simulink model "power_PVarray_grid_det_LVRT"  (Simulink 8.7)
settings: Solver=FixedStepDiscrete  SolverMode=SingleTasking  StartTime=0.0  StopTime=1.666666  RelTol=1e-3
PreLoadFcn:
  | Ts_Power=1e-6;
  | Ts_Control=100e-6;
undefined symbols (not defined in the file): D1, Delta, DiscIntNeverNeededParam, sigbuilder_block
libraries: powerlib x30, powerlib_meascontrol x17, simulink x6, re_lib x1
(part 1 of 2)
Description:
  | Copyright 2008-2016 The MathWorks, Inc.
settings Model: Creator=MathWorks  LastModifiedBy=jherna4  SimulationMode=accelerator
settings DataIOCC: SignalLoggingSaveFormat=ModelDataLogs  SignalLogging=off  DSMLogging=off
settings OptimizationCC: ExpressionDepthLimit=2147483647
settings DebuggingCC: SolverPrmCheckMsg=warning  FcnCallInpInsideContextMsg=EnableAllAsWarning  StateNameClashWarn=warning
settings GRTTargetCC: CombineOutputUpdateFcns=off  GRTInterface=on
settings ConfigComp: CovModelRefEnable=off  CovSFcnEnable=off

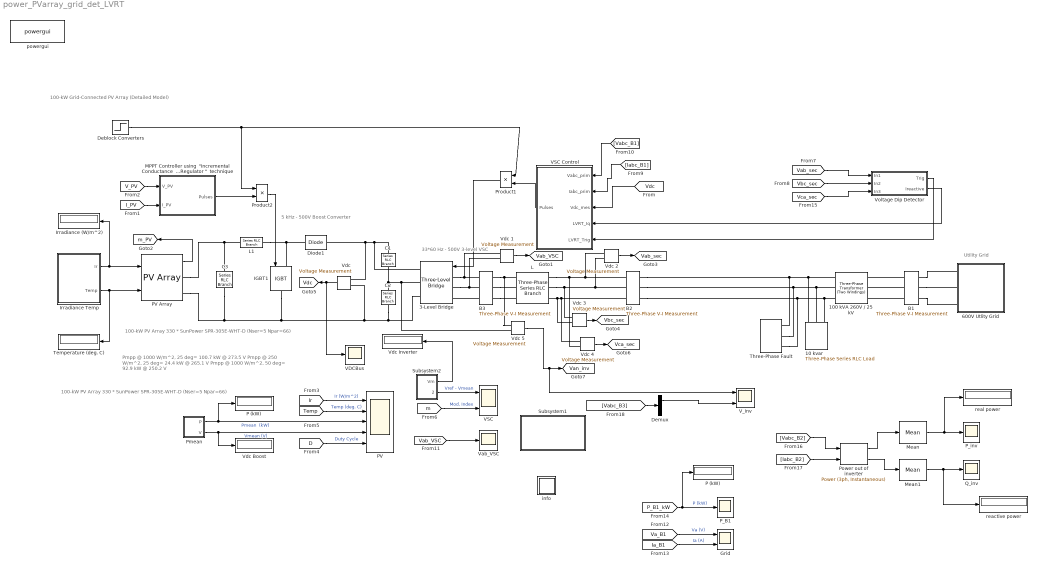
== system power_PVarray_grid_det_LVRT ==
  note: 5 kHz - 500V
      | Boost Converter
  note: 33*60 Hz - 500V
      | 3-level VSC
  note: 100-kW Grid-Connected PV Array (Detailed Model)
  note: Utility Grid
  note: Pmpp @ 1000 W/m^2, 25 deg= 100.7 kW @ 273.5 V
      | Pmpp @  250 W/m^2, 25 deg= 24.4  kW @ 265.1 V
      | Pmpp @ 1000 W/m^2, 50 deg= 92.9  kW @ 250.2 V
  note: 100-kW  PV Array
      | 330 * SunPower SPR-305E-WHT-D  (Nser=5 Npar=66)
  note: 100-kW  PV Array
      | 330 * SunPower SPR-305E-WHT-D  (Nser=5 Npar=66)
  10 kvar : powerlib/Elements/Three-Phase Series RLC Load  LConnTagsString=A|B|C  Configuration=Y (grounded)  NominalVoltage=240  Vabc=[1e3 1e3 1e3]  Vabcp=[1e3 1e3 1e3]  NominalFrequency=60  UnbalancedPower=off  ActivePower=10e3/100  InductivePower=0  CapacitivePower=10e3  Pabc=[10e3 9e3 11e3]  QLabc=[100 90 110]  QCabc=[100 90 110]  Pabcp=[10e3 9e3 11e3]  QLabcp=[100 90 110]  QCabcp=[100 90 110]  Measurements=None  LoadType=constant Z
  100 kVA 260V / 25 kV : powerlib/Elements/Three-Phase Transformer (Two Windings)  Winding1Connection=Yg  Winding2Connection=Delta (D1)  CoreType=Three single-phase transformers  SetSaturation=off  Hysteresis=off  DataFile='hysteresis'  SetInitialFlux=off  Measurements=None  UNITS=pu  NominalPower=[100e3 , 60 ]  Winding1=[ 25e3 , 0.001 , 0.03 ]  Winding2=[ 260 , 0.001 , 0.03 ]  Rm=500  Lm=500  L0=0.5  Saturation=[ 0,0 ; 0.0024,1.2 ; 1.0,1.52 ]  InitialFluxes=[ 0.8 , -0.8 , 0.7 ]  MoreParameters=off  BreakLoop=off  DataType=off  TransfoNumber=0
  3-Level Bridge : powerlib/Power Electronics/Three-Level Bridge  Arms=3  SnubberResistance=1e6  SbubberCapacitance=inf  Device=IGBT / Diodes  Ron=0.2e-3  ForwardVoltages="[  0  0 ]"  Measurements=None
  600V Utlity Grid : Subsystem
      mask Display: image(imread('grid.jpg'))
  B1 : powerlib/Measurements/Three-Phase V-I Measurement  VoltageMeasurement=phase-to-ground  SetLabelV=on  LabelV=Vabc_B1  Vpu=off  VpuLL=off  CurrentMeasurement=yes  SetLabelI=on  LabelI=Iabc_B1  Ipu=off  Pbase=100e6  Vbase=500e3  OutputType=Magnitude  PhasorSimulation=off  PSBequivalent=0
  B2 : powerlib/Measurements/Three-Phase V-I Measurement  VoltageMeasurement=phase-to-ground  SetLabelV=on  LabelV=Vabc_B2  Vpu=off  VpuLL=off  CurrentMeasurement=yes  SetLabelI=on  LabelI=Iabc_B2  Ipu=off  Pbase=100e6  Vbase=500e3  OutputType=Magnitude  PhasorSimulation=off  PSBequivalent=0
  B3 : powerlib/Measurements/Three-Phase V-I Measurement  VoltageMeasurement=phase-to-ground  SetLabelV=on  LabelV=Vabc_B3  Vpu=off  VpuLL=off  CurrentMeasurement=yes  SetLabelI=on  LabelI=Iabc_B3  Ipu=off  Pbase=100e6  Vbase=500e3  OutputType=Magnitude  PhasorSimulation=off  PSBequivalent=0
  C1 : powerlib/Elements/Series RLC Branch  LConnTagsString=__new0  RConnTagsString=__new0  BranchType=C  Resistance=1.0  Inductance=1.0  SetiL0=off  InitialCurrent=0  Capacitance=12000e-06  Setx0=off  InitialVoltage=0  Measurements=None
  C2 : powerlib/Elements/Series RLC Branch  LConnTagsString=__new0  RConnTagsString=__new0  BranchType=C  Resistance=1.0  Inductance=1.0  SetiL0=off  InitialCurrent=0  Capacitance=12000e-06  Setx0=off  InitialVoltage=0  Measurements=None
  C3 : powerlib/Elements/Series RLC Branch  LConnTagsString=__new0  RConnTagsString=__new0  BranchType=C  Resistance=1.0  Inductance=1.0  SetiL0=off  InitialCurrent=0  Capacitance=100e-6  Setx0=off  InitialVoltage=0  Measurements=Branch voltage
  Deblock Converters : Step  Time=0.05  SampleTime=0
  Demux : Demux  Outputs=3
  Diode1 : powerlib/Power Electronics/Diode  Ron=1e-4  Lon=0  Vf=0  IC=0  UseSnubber=off  Rs=inf  Cs=inf  Measurements=off
  Grid : Scope  NumInputPorts=2
  IGBT1 : powerlib/Power Electronics/IGBT  Ron=0.001  Lon=0  Vf=0  Tf=0  Tt=0  IC=0  Rs=1e5  Cs=inf  Measurements=off
  Irradiance (W/m^2) : Display
      settings: Format=bank  Decimation=1000
  Irradiance Temp : Subsystem  Tag=STV Subsys  LoadFcn=sigbuilder_block('load');  StartFcn=sigbuilder_block('start');  StopFcn=sigbuilder_block('stop');  ClipboardFcn=sigbuilder_block('clipboard');  mask(Sigbuilder block){}
      mask help: Sigbuilder GUI
      mask init:
      | if ~strcmp(get_param(bdroot(gcbh),'SimulationStatus'),'stopped') tuvar = sigbuilder_block('maskInit'); end
      settings: CopyFcn=sigbuilder_block('copy');  DeleteFcn=sigbuilder_block('delete');  ModelCloseFcn=sigbuilder_block('modelClose');  PreSaveFcn=sigbuilder_block('preSave');  PauseFcn=sigbuilder_block('pause')  ContinueFcn=sigbuilder_block('continue')  NameChangeFcn=sigbuilder_block('namechange');  OpenFcn=sigbuilder_block('open',[6 30 1428 682.5 ]);  CloseFcn=sigbuilder_block('close');
      mask Display: plot(0,0,100,100,[10,10,40,40,10],[80,20,20,80,80],[40,10],[50,50], [40,27,10],[65,72,56],[40,25,25,10],[28,28,43,43]);
  L : powerlib/Elements/Three-Phase Series RLC Branch  LConnTagsString=A|B|C  RConnTagsString=A|B|C  BranchType=RL  Resistance=500e-6*377/50/2  Inductance=500e-6/2  Capacitance=inf  Measurements=None
  L1 : powerlib/Elements/Series RLC Branch  LConnTagsString=__new0  RConnTagsString=__new0  BranchType=RL  Resistance=0.005  Inductance=5e-3  SetiL0=off  InitialCurrent=0  Capacitance=1e-6  Setx0=off  InitialVoltage=0  Measurements=None
  "MPPT Controller using  \"Incremental Conductance  + Integral Regulator \"  technique " : Subsystem  mask(Boost Control - MPPT){fc=5000, T_MPPT=200e-6, Dinit=0.5}
      mask prompts: fc "PWM switching frequency (Hz)"; T_MPPT "Time window used by MPPT control (s)"; Dinit "Initial value of duty cycle"
  Mean : powerlib_meascontrol/Measurements/Mean  Freq=60  Vinit=0  Ts=Ts_Power
  Mean1 : powerlib_meascontrol/Measurements/Mean  Freq=60  Vinit=0  Ts=Ts_Power
  P (kW) : Display
      settings: Format=bank  Decimation=2000
  "P (kW) " : Display
      settings: Format=bank  Decimation=2000
  PV : Scope  NumInputPorts=5
  PV Array : re_lib/Solar/PV Array  Npar=66  Nser=5  PlotType=array @ 1000 W/m2 & specified temperatures  S_vec="[ 1000  250 ]"  Temp_C_vec="[0 25 50  ]"  ModuleName=SunPower SPR-305E-WHT-D  PlotWhenSelected=off  Pm=305.226  Ncell=96  Voc=64.2  Isc=5.96  Vm=54.7  Im=5.58  beta_Voc_pc=-0.27269  alpha_Isc_pc=0.061745  beta_Voc=-0.17507  alpha_Isc=0.00368  IL=6.0092  I0=6.3014e-12  nI=0.94504  Rsh=269.5934  Rs=0.37152  BAL=on  Tc=Tc  Tfilter=Tc
  P_B1 : Scope
  P_inv : Scope
  Pmean : Subsystem
  Power out of inverter : powerlib_meascontrol/Measurements/Power (3ph, Instantaneous)
  Product1 : Product  RndMeth=Zero
  Product2 : Product  RndMeth=Zero
  Q_inv : Scope
  Subsystem1 : Subsystem
      mask Display: disp('Open this block\nto display additional \nscopes & measurements')
  Subsystem2 : Subsystem
  Temperature (deg. C) : Display
      settings: Format=bank  Decimation=1000
  Three-Phase Fault : powerlib/Elements/Three-Phase Fault  InitialStates=0  FaultA=on  FaultB=on  FaultC=on  GroundFault=on  SwitchTimes="[90/60  100/60]"  External=off  SwitchStatus=NaN  FaultResistance=0.025  GroundResistance=0.01  SnubberResistance=1e6  SnubberCapacitance=inf  Measurements=None
  VDCBus : Scope
  VSC : Scope  NumInputPorts=2
  VSC Control : Subsystem  mask(VSC Main Controller){nom=[ 100e3  60 ], Vnom=[ 25e3 260 ], Vnom_dc=500, RLxfo=[0.002  0.06 ], RLchoke=[2e-3  250e-6  ], K_VDCreg=[7  800], K_Ireg=[0.3 20], Ts=Ts_Control}
      mask prompts: nom "Nominal power and frequency [ Pnom(VA)  Fnom(Hz) ]:"; Vnom "Nominal primary and secondary voltages (Vrms LL) [ Vnom_prim   Vnom_sec ]:"; Vnom_dc "Nominal DC bus voltage (V):"; RLxfo "Total transformer leakage impedance (pu/Pnom) [ Rxfo  Lxf ]"; RLchoke "Choke impedance [ R(ohm) L(H) ]"; K_VDCreg "VDC regultator gains [ Kp  Ki ]:"; K_Ireg "Current regulator gains [ Kp  Ki ]:"; Ts "Sample time"
      mask init:
      | Pnom=nom(1);
      | Fnom=nom(2);
      | Vnom_prim=Vnom(1);
      | Vnom_sec=Vnom(2);
      | Zbase=Vnom_sec^2/Pnom;
      | Rtot_pu=RLxfo(1) + RLchoke(1)/Zbase;
      | Ltot_pu=RLxfo(2) + RLchoke(2)/(Zbase/(2*pi*Fnom));
      | Kp_VDCreg=K_VDCreg(1);
      | Ki_VDCreg=K_VDCreg(2);
      | Kp_Ireg=K_Ireg(1);
      | Ki_Ireg=K_Ireg(2);
      | Vdc_ref=Vnom_dc;
      | % Used to determine initial value of Boost Control (MPPT)
      | assignin('base','Vdc_ref_Inv',Vdc_ref);
  "V_inv " : Scope  NumInputPorts=2
  Vab_VSC : Scope
  Vdc {,1..5} (6 alike) : powerlib/Measurements/Voltage Measurement  Tag=PoWeRsYsTeMmEaSuReMeNt  PhasorSimulation=off  OutputType=Magnitude  PSBequivalent=0
  Vdc Boost : Display
      settings: Format=bank  Decimation=2000
  Vdc Inverter : Display
      settings: Format=bank  Decimation=2000
  Voltage Dip Detector : Subsystem
  info : Subsystem
      settings: OpenFcn=showdemo(bdroot(gcb))
      mask Display: disp('?')
  powergui : powerlib/powergui  Priority=1  SimulationMode=Discrete  SolverType=Tustin/Backward Euler (TBE)  SampleTime=Ts_Power  frequency=60  SPID=off  DisableSnubberDevices=off  DisableRonSwitches=off  DisableVfSwitches=off  SwTol=0  DisplayEquations=off  Interpol=off  ExternalGateDelay=off  methode=off  Ts=0  FunctionMessages=off  echomessages=off  HookPort=off  EnableUseOfTLC=off  x0status=blocks  frequencyindice=0  Pbase=100e6  ErrMax=1e-4  Iterations=50  UnitsV=kV  UnitsW=MW  buscounter=0  RestoreLinks=warning  ResistiveCurrentMeasurement=off  Frange=[0:2:500]  Ylog=off  Xlog=on  ShowGrid=off  save=off  variable=ZData  structure=0  ZoomFFT=on  StartTime=0.0  cycles=1  DisplayStyle=1  fundamental=60  FreqAxis=off  MaxFrequency=1000  frequencyindicesteady=1  RmsSteady=1  display=off
  reactive power : Display
  real power : Display
  tag scope: Vab_VSC=global, Vab_sec=global, Van_inv=global, Vbc_sec=global, Vca_sec=global, Vdc=global, m_PV=global
  wires:
  "Vdc "/1 -> VDCBus/1, [Vdc]
  Product2/1 -> IGBT1/1
  "MPPT Controller using  \"Incremental Conductance  + Integral Regulator \"  technique "/1(Pulses) -> Product2/2
  Deblock Converters/1 -> Product2/1, Product1/1
  [Vabc_B1] -> VSC Control/1(Vabc_prim)
  [Iabc_B1] -> VSC Control/2(Iabc_prim)
  [Vdc] -> VSC Control/3(Vdc_mes)
  VSC Control/1(Pulses) -> Product1/2
  Product1/1 -> 3-Level Bridge/1
  [I_PV] -> "MPPT Controller using  \"Incremental Conductance  + Integral Regulator \"  technique "/2(I_PV)
  [V_PV] -> "MPPT Controller using  \"Incremental Conductance  + Integral Regulator \"  technique "/1(V_PV)
  Pmean/1(P) -> "P (kW) "/1, PV/3  "Pmean  (kW)"
  [m] -> VSC/2  "Mod. Index"
  Vdc 1/1 -> [Vab_VSC]
  [Vab_VSC] -> Vab_VSC/1
  [Ia_B1] -> Grid/2  "Ia (A)"
  [Va_B1] -> Grid/1  "Va (V)"
  [P_B1_kW] -> P_B1/1, P (kW)/1  "P (kW)"
  Pmean/2(V) -> Vdc Boost/1, PV/4  "Vmean (V)"
  Subsystem2/2(VrVm) -> VSC/1  "Vref - Vmean"
  Subsystem2/1(Vm) -> Vdc Inverter/1
  PV Array/1 -> [m_PV]
  Irradiance Temp/1(Ir) -> PV Array/1, Irradiance (W/m^2)/1
  Irradiance Temp/2(Temp) -> PV Array/2, Temperature (deg. C)/1
  [D] -> PV/5  "Duty Cycle"
  [Temp] -> PV/2  "Temp (deg. C)"
  [Ir] -> PV/1  "Ir (W/m^2)"
  Vdc 2/1 -> [Vab_sec]
  Vdc 3/1 -> [Vbc_sec]
  Vdc 4/1 -> [Vca_sec]
  [Vab_sec] -> Voltage Dip Detector/1(In1)
  [Vbc_sec] -> Voltage Dip Detector/2(In2)
  [Vca_sec] -> Voltage Dip Detector/3(In3)
  [Vabc_B2] -> Power out of inverter/1
  [Iabc_B2] -> Power out of inverter/2
  Power out of inverter/1 -> Mean/1
  Power out of inverter/2 -> Mean1/1
  Mean/1 -> real power/1, P_inv/1
  Mean1/1 -> reactive power/1, Q_inv/1
  Voltage Dip Detector/1(Trig) -> VSC Control/5(LVRT_Trig)
  Voltage Dip Detector/2(Ireactive) -> VSC Control/4(LVRT_Iq)
  Vdc 5/1 -> "V_inv "/1, [Van_inv]
  [Vabc_B3] -> Demux/1
  Demux/1 -> "V_inv "/2
  connections:
  C1/LConn1 -- 3-Level Bridge/RConn1 -- Diode1/RConn1 -- "Vdc "/LConn1
  L1/RConn1 -- Diode1/LConn1 -- IGBT1/LConn1
  3-Level Bridge/RConn3 -- C2/RConn1 -- "Vdc "/LConn2 -- IGBT1/RConn1 -- PV Array/RConn2 -- C3/RConn1
  3-Level Bridge/LConn1 -- B3/LConn1 -- Vdc 1/LConn1
  3-Level Bridge/LConn2 -- B3/LConn2 -- Vdc 1/LConn2
  L/RConn1 -- B2/LConn1 -- Vdc 2/LConn1 -- Vdc 4/LConn2
  L/RConn2 -- B2/LConn2 -- Vdc 2/LConn2 -- Vdc 3/LConn1
  Three-Phase Fault/LConn3 -- B2/RConn3 -- 100 kVA 260V / 25 kV/RConn3 -- 10 kvar/LConn3
  B1/LConn1 -- 100 kVA 260V / 25 kV/LConn1
  B1/LConn2 -- 100 kVA 260V / 25 kV/LConn2
  B1/LConn3 -- 100 kVA 260V / 25 kV/LConn3
  C2/LConn1 -- Vdc 5/LConn2 -- 3-Level Bridge/RConn2 -- C1/RConn1
  C3/LConn1 -- PV Array/RConn1 -- L1/LConn1
  B1/RConn2 -- 600V Utlity Grid/LConn2
  B1/RConn1 -- 600V Utlity Grid/LConn1
  B1/RConn3 -- 600V Utlity Grid/LConn3
  Three-Phase Fault/LConn1 -- 100 kVA 260V / 25 kV/RConn1 -- 10 kvar/LConn1 -- B2/RConn1
  Three-Phase Fault/LConn2 -- B2/RConn2 -- 100 kVA 260V / 25 kV/RConn2 -- 10 kvar/LConn2
  L/RConn3 -- B2/LConn3 -- Vdc 4/LConn1 -- Vdc 3/LConn2
  B3/RConn1 -- Vdc 5/LConn1 -- L/LConn1
  B3/RConn2 -- L/LConn2
  B3/LConn3 -- 3-Level Bridge/LConn3
  B3/RConn3 -- L/LConn3

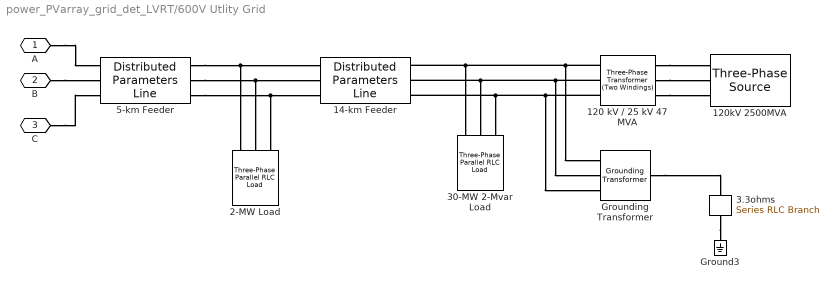
== system power_PVarray_grid_det_LVRT/600V Utlity Grid ==
  120 kV / 25 kV 47 MVA : powerlib/Elements/Three-Phase Transformer (Two Windings)  Winding1Connection=Yg  Winding2Connection=Delta (D1)  CoreType=Three single-phase transformers  SetSaturation=off  Hysteresis=off  DataFile='basic_model'  SetInitialFlux=off  Measurements=None  UNITS=pu  NominalPower=[47e6 60 ]  Winding1="[ 120e3  0.08/30   0.08 ]"  Winding2="[ 25e3  0.08/30  0.08]"  Rm=500  Lm=500  L0=0.5  Saturation="[ 0,0  ;  0.005,1.2  ;  1.0,1.4 ]"  InitialFluxes=[ 0.8 , -0.8 , 0.7 ]  MoreParameters=off  BreakLoop=off  DataType=off  TransfoNumber=0
  120kV 2500MVA : powerlib/Electrical Sources/Three-Phase Source  InternalConnection=Yg  VoltagePhases=off  Voltage=120e3  PhaseAngle=0  Voltage_phases=[25e3 25e3 25e3]/sqrt(3)  PhaseAngles_phases=[0 -120 +120]  Frequency=60  NonIdealSource=on  SpecifyImpedance=on  Resistance=0.8929  Inductance=16.58e-3  ShortCircuitLevel=2500e6  BaseVoltage=120e3  XRratio=7  BusType=swing  Pref=0  Qref=0  Prefabc=[10e3, 10e3, 10e3]  Qrefabc=[0, 0, 0]  Qmin=-inf  Qmax=inf
  14-km Feeder : powerlib/Elements/Distributed Parameters Line  Phases=3  Frequency=60  Resistance=[0.1153 0.413]  Inductance=[1.05e-3 3.32e-3]  Capacitance=[11.33e-009 5.01e-009]  Length=14  x1=[-5.8e-05 -3.07268501543022e-09 0 0;-5.7e-05 -3.07225125790422e-09 0 0;-5.6e-05 -3.07181706374279e-09 0 0;-5.5e-05 -3.07138243300766e-09 0 0;-5.4e-05 -3.07094736576058e-09 0 0;-5.3e-05 -3.0705118620634e-09 0 0;-5.2e-05 -3.070075921978e-09 0 0;-5.1e-05 -3.06963954556634e-09 0 0;-5e-05 -3.06920273289045e-09 0 0;-4.9e-05 -3.0687654840124e-09 -3790.73537143814 -24061.4134110798;-4.8e-05 -3.06832779899434e-09 -3781.66416312612 -24062.8407747816;-4.7e-05 -3.06788967789847e-09 -3772.59241735528 -24064.264718617;-4.6e-05 -3.06745112078705e-09 -3763.52013541492 -24065.6852423838;-4.5e-05 -3.06701212772242e-09 -3754.44731859442 -24067.10234588;-4.4e-05 -3.06657269876697e-09 -3745.37396818323 -24068.5160289042;-4.3e-05 -3.06613283398315e-09 -3736.30008547086 -24069.9262912555;-4.2e-05 -3.06569253343347e-09 -3727.22567174693 -24071.3331327335;-4.1e-05 -3.06525179718052e-09 -3718.15072830111 -24072.7365531382;-4e-05 -3.06481062528692e-09 -3709.07525642314 -24074.1365522702;-3.9e-05 -3.06436901781538e-09 -3699.99925740287 -24075.5331299305;-3.8e-05 -3.06392697482867e-09 -3690.92273253018 -24076.9262859206;-3.7e-05 -3.0634844963896e-09 -3681.84568309506 -24078.3160200426;-3.6e-05 -3.06304158256106e-09 -3672.76811038756 -24079.7023320988;-3.5e-05 -3.06259823340601e-09 -3663.6900156978 -24081.0852218923;-3.4e-05 -3.06215444898744e-09 -3654.61140031598 -24082.4646892266;-3.3e-05 -3.06171022936843e-09 -3645.53226553238 -24083.8407339055;-3.2e-05 -3.06126557461212e-09 -3636.45261263734 -24085.2133557336;-3.1e-05 -3.0608204847817e-09 -3627.37244292129 -24086.5825545157;-3e-05 -3.06037495994043e-09 -3618.29175767471 -24087.9483300573;-2.9e-05 -3.05992900015163e-09 -3609.21055818818 -24089.3106821641;-2.8e-05 -3.05948260547867e-09 -3600.12884575234 -24090.6696106428;-2.7e-05 -3.059035775985e-09 -3591.04662165791 -24092.0251153;-2.6e-05 -3.05858851173413e-09 -3581.96388719566 -24093.3771959431;-2.5e-05 -3.05814081278961e-09 -3572.88064365646 -24094.72585238;-2.4e-05 -3.05769267921509e-09 -3563.79689233123 -24096.071084419;-2.3e-05 -3.05724411107425e-09 -3554.712634511 -24097.412891869;-2.2e-05 -3.05679510843083e-09 -3545.62787148682 -24098.7512745391;-2.1e-05 -3.05634567134866e-09 -3536.54260454984 -24100.0862322393;-2e-05 -3.05589579989161e-09 -3527.45683499129 -24101.4177647797;-1.9e-05 -3.05544549412361e-09 -3518.37056410246 -24102.7458719712;-1.8e-05 -3.05499475410866e-09 -3509.2837931747 -24104.0705536249;-1.7e-05 -3.05454357991083e-09 -3500.19652349946 -24105.3918095526;-1.6e-05 -3.05409197159424e-09 -3491.10875636822 -24106.7096395666;-1.5e-05 -3.05363992922306e-09 -3482.02049307258 -24108.0240434795;-1.4e-05 -3.05318745286155e-09 -3472.93173490417 -24109.3350211046;-1.3e-05 -3.05273454257401e-09 -3463.8424831547 -24110.6425722555;-1.2e-05 -3.05228119842481e-09 -3454.75273911597 -24111.9466967463;-1.1e-05 -3.05182742047839e-09 -3445.66250407983 -24113.2473943918;-1e-05 -3.05137320879922e-09 -3436.5717793382 -24114.5446650071;-9e-06 -3.05091856345187e-09 -3427.48056618309 -24115.8385084078;-8e-06 -3.05046348450096e-09 -3418.38886590654 -24117.12892441;-7e-06 -3.05000797201115e-09 -3409.2966798007 -24118.4159128303;-6e-06 -3.04955202604718e-09 -3400.20400915777 -24119.6994734858;-5e-06 -3.04909564667387e-09 -3391.11085527002 -24120.9796061942;-4e-06 -3.04863883395606e-09 -3382.01721942979 -24122.2563107734;-3e-06 -3.04818158795869e-09 -3372.92310292949 -24123.529587042;-2e-06 -3.04772390874673e-09 -3363.82850706159 -24124.7994348191;-1e-06 -3.04726579638523e-09 -3354.73343311865 -24126.0658539241]  x2=[-5.8e-05 -3.21435514712151e-09 0 0;-5.7e-05 -3.21386287362357e-09 0 0;-5.6e-05 -3.21337014336404e-09 0 0;-5.5e-05 -3.21287695641295e-09 0 0;-5.4e-05 -3.21238331284039e-09 0 0;-5.3e-05 -3.21188921271652e-09 0 0;-5.2e-05 -3.21139465611156e-09 0 0;-5.1e-05 -3.2108996430958e-09 0 0;-5e-05 -3.2104041737396e-09 0 0;-4.9e-05 -3.20990824811336e-09 -3379.39243175417 -24244.0512711511;-4.8e-05 -3.20941186628758e-09 -3370.25239982314 -24245.3235492432;-4.7e-05 -3.20891502833279e-09 -3361.11188890409 -24246.5923815342;-4.6e-05 -3.20841773431962e-09 -3351.97090029607 -24247.8577678435;-4.5e-05 -3.20791998431873e-09 -3342.82943529824 -24249.1197079916;-4.4e-05 -3.20742177840087e-09 -3333.6874952098 -24250.3782017989;-4.3e-05 -3.20692311663684e-09 -3324.54508133001 -24251.6332490867;-4.2e-05 -3.20642399909752e-09 -3315.40219495823 -24252.8848496765;-4.1e-05 -3.20592442585384e-09 -3306.25883739385 -24254.1330033905;-4e-05 -3.2054243969768e-09 -3297.11500993636 -24255.3777100513;-3.9e-05 -3.20492391253747e-09 -3287.9707138853 -24256.618969482;-3.8e-05 -3.20442297260698e-09 -3278.82595054026 -24257.8567815062;-3.7e-05 -3.20392157725652e-09 -3269.68072120094 -24259.0911459479;-3.6e-05 -3.20341972655734e-09 -3260.53502716707 -24260.3220626318;-3.5e-05 -3.20291742058079e-09 -3251.38886973846 -24261.5495313829;-3.4e-05 -3.20241465939823e-09 -3242.24225021497 -24262.7735520267;-3.3e-05 -3.20191144308114e-09 -3233.09516989656 -24263.9941243892;-3.2e-05 -3.20140777170102e-09 -3223.94763008321 -24265.2112482971;-3.1e-05 -3.20090364532946e-09 -3214.79963207501 -24266.4249235773;-3e-05 -3.2003990640381e-09 -3205.65117717209 -24267.6351500573;-2.9e-05 -3.19989402789867e-09 -3196.50226667464 -24268.8419275652;-2.8e-05 -3.19938853698293e-09 -3187.35290188293 -24270.0452559294;-2.7e-05 -3.19888259136273e-09 -3178.2030840973 -24271.2451349789;-2.6e-05 -3.19837619110997e-09 -3169.05281461812 -24272.4415645432;-2.5e-05 -3.19786933629662e-09 -3159.90209474587 -24273.6345444522;-2.4e-05 -3.19736202699473e-09 -3150.75092578105 -24274.8240745364;-2.3e-05 -3.19685426327638e-09 -3141.59930902426 -24276.0101546268;-2.2e-05 -3.19634604521375e-09 -3132.44724577615 -24277.1927845547;-2.1e-05 -3.19583737287906e-09 -3123.29473733743 -24278.371964152;-2e-05 -3.19532824634461e-09 -3114.14178500886 -24279.5476932513;-1.9e-05 -3.19481866568275e-09 -3104.9883900913 -24280.7199716854;-1.8e-05 -3.19430863096591e-09 -3095.83455388564 -24281.8887992877;-1.7e-05 -3.19379814226657e-09 -3086.68027769285 -24283.054175892;-1.6e-05 -3.19328719965729e-09 -3077.52556281396 -24284.2161013328;-1.5e-05 -3.19277580321069e-09 -3068.37041055005 -24285.3745754449;-1.4e-05 -3.19226395299944e-09 -3059.21482220227 -24286.5295980637;-1.3e-05 -3.19175164909629e-09 -3050.05879907184 -24287.6811690249;-1.2e-05 -3.19123889157404e-09 -3040.90234246004 -24288.8292881651;-1.1e-05 -3.19072568050559e-09 -3031.74545366819 -24289.9739553209;-1e-05 -3.19021201596385e-09 -3022.5881339977 -24291.1151703297;-9e-06 -3.18969789802184e-09 -3013.43038475003 -24292.2529330293;-8e-06 -3.18918332675262e-09 -3004.2722072267 -24293.387243258;-7e-06 -3.18866830222933e-09 -2995.11360272928 -24294.5181008546;-6e-06 -3.18815282452516e-09 -2985.95457255943 -24295.6455056583;-5e-06 -3.18763689371337e-09 -2976.79511801884 -24296.769457509;-4e-06 -3.18712050986728e-09 -2967.63524040928 -24297.8899562469;-3e-06 -3.1866036730603e-09 -2958.47494103256 -24299.0070017128;-2e-06 -3.18608638336587e-09 -2949.31422119058 -24300.1205937478;-1e-06 -3.18556864085751e-09 -2940.15308218527 -24301.2307321938]  x3=[-5.8e-05 -1.41208605432097e-11 0 0;-5.7e-05 -1.41218449859166e-11 0 0;-5.6e-05 -1.41228274215944e-11 0 0;-5.5e-05 -1.41238078501035e-11 0 0;-5.4e-05 -1.41247862713045e-11 0 0;-5.3e-05 -1.41257626850583e-11 0 0;-5.2e-05 -1.41267370912263e-11 0 0;-5.1e-05 -1.41277094896699e-11 0 0;-5e-05 -1.41286798802508e-11 0 0;-4.9e-05 -1.41296482628313e-11 -23.5442852816691 -155.681480348964;-4.8e-05 -1.41306146372736e-11 -23.4855930745795 -155.69034527229;-4.7e-05 -1.41315790034405e-11 -23.4268975296635 -155.699188068545;-4.6e-05 -1.41325413611948e-11 -23.3681986552628 -155.708008736473;-4.5e-05 -1.41335017103998e-11 -23.30949645972 -155.716807274821;-4.4e-05 -1.4134460050919e-11 -23.2507909513778 -155.725583682338;-4.3e-05 -1.41354163826162e-11 -23.1920821385798 -155.734337957776;-4.2e-05 -1.41363707053555e-11 -23.1333700296696 -155.743070099892;-4.1e-05 -1.41373230190013e-11 -23.0746546329917 -155.751780107444;-4e-05 -1.41382733234182e-11 -23.0159359568907 -155.760467979195;-3.9e-05 -1.41392216184711e-11 -22.9572140097119 -155.76913371391;-3.8e-05 -1.41401679040253e-11 -22.8984887998011 -155.777777310356;-3.7e-05 -1.41411121799463e-11 -22.8397603355043 -155.786398767307;-3.6e-05 -1.41420544460999e-11 -22.7810286251682 -155.794998083535;-3.5e-05 -1.41429947023522e-11 -22.7222936771398 -155.803575257821;-3.4e-05 -1.41439329485695e-11 -22.6635554997668 -155.812130288943;-3.3e-05 -1.41448691846185e-11 -22.6048141013971 -155.820663175687;-3.2e-05 -1.41458034103661e-11 -22.5460694903792 -155.829173916839;-3.1e-05 -1.41467356256796e-11 -22.4873216750621 -155.837662511191;-3e-05 -1.41476658304265e-11 -22.428570663795 -155.846128957535;-2.9e-05 -1.41485940244745e-11 -22.3698164649278 -155.854573254669;-2.8e-05 -1.41495202076918e-11 -22.3110590868108 -155.862995401392;-2.7e-05 -1.41504443799467e-11 -22.2522985377947 -155.871395396508;-2.6e-05 -1.41513665411079e-11 -22.1935348262308 -155.879773238822;-2.5e-05 -1.41522866910443e-11 -22.1347679604706 -155.888128927143;-2.4e-05 -1.41532048296251e-11 -22.0759979488662 -155.896462460285;-2.3e-05 -1.41541209567199e-11 -22.0172247997702 -155.904773837063;-2.2e-05 -1.41550350721984e-11 -21.9584485215356 -155.913063056296;-2.1e-05 -1.41559471759308e-11 -21.8996691225157 -155.921330116806;-2e-05 -1.41568572677874e-11 -21.8408866110644 -155.929575017417;-1.9e-05 -1.41577653476388e-11 -21.782100995536 -155.937797756958;-1.8e-05 -1.41586714153561e-11 -21.7233122842853 -155.94599833426;-1.7e-05 -1.41595754708103e-11 -21.6645204856674 -155.954176748158;-1.6e-05 -1.41604775138731e-11 -21.6057256080381 -155.962332997489;-1.5e-05 -1.41613775444163e-11 -21.5469276597533 -155.970467081095;-1.4e-05 -1.41622755623119e-11 -21.4881266491695 -155.978578997819;-1.3e-05 -1.41631715674323e-11 -21.4293225846437 -155.986668746508;-1.2e-05 -1.41640655596501e-11 -21.3705154745333 -155.994736326013;-1.1e-05 -1.41649575388384e-11 -21.311705327196 -156.002781735187;-1e-05 -1.41658475048702e-11 -21.2528921509901 -156.010804972886;-9e-06 -1.41667354576193e-11 -21.1940759542742 -156.018806037971;-8e-06 -1.41676213969592e-11 -21.1352567454075 -156.026784929304;-7e-06 -1.41685053227642e-11 -21.0764345327495 -156.034741645751;-6e-06 -1.41693872349087e-11 -21.0176093246601 -156.042676186182;-5e-06 -1.41702671332672e-11 -20.9587811294996 -156.050588549468;-4e-06 -1.41711450177147e-11 -20.899949955629 -156.058478734485;-3e-06 -1.41720208881264e-11 -20.8411158114093 -156.066346740112;-2e-06 -1.4172894744378e-11 -20.7822787052023 -156.074192565231;-1e-06 -1.41737665863451e-11 -20.72343864537 -156.082016208726]  x4=[-5.8e-05 6.64255961640974e-12 0 0;-5.7e-05 6.64505542156155e-12 0 0;-5.6e-05 6.64755028230278e-12 0 0;-5.5e-05 6.65004419827886e-12 0 0;-5.4e-05 6.65253716913536e-12 0 0;-5.3e-05 6.65502919451797e-12 0 0;-5.2e-05 6.6575202740725e-12 0 0;-5.1e-05 6.66001040744494e-12 0 0;-5e-05 6.66249959428136e-12 0 0;-4.9e-05 6.66498783422801e-12 -1.3558131993987 -2.1529826150637;-4.8e-05 6.66747512693124e-12 -1.35500144774826 -2.1534935915926;-4.7e-05 6.66996147203756e-12 -1.3541895035219 -2.15400426206203;-4.6e-05 6.67244686919361e-12 -1.35337736683501 -2.15451462639942;-4.5e-05 6.67493131804615e-12 -1.35256503780302 -2.15502468453224;-4.4e-05 6.67741481824208e-12 -1.35175251654137 -2.15553443638798;-4.3e-05 6.67989736942846e-12 -1.35093980316553 -2.15604388189421;-4.2e-05 6.68237897125244e-12 -1.35012689779103 -2.15655302097852;-4.1e-05 6.68485962336135e-12 -1.34931380053338 -2.15706185356855;-4e-05 6.68733932540261e-12 -1.34850051150815 -2.15757037959198;-3.9e-05 6.68981807702382e-12 -1.34768703083092 -2.15807859897655;-3.8e-05 6.69229587787269e-12 -1.34687335861731 -2.15858651165002;-3.7e-05 6.69477272759707e-12 -1.34605949498296 -2.15909411754021;-3.6e-05 6.69724862584493e-12 -1.34524544004353 -2.15960141657497;-3.5e-05 6.69972357226441e-12 -1.34443119391473 -2.1601084086822;-3.4e-05 6.70219756650375e-12 -1.34361675671227 -2.16061509378986;-3.3e-05 6.70467060821134e-12 -1.3428021285519 -2.16112147182592;-3.2e-05 6.70714269703572e-12 -1.34198730954941 -2.16162754271843;-3.1e-05 6.70961383262554e-12 -1.34117229982059 -2.16213330639546;-3e-05 6.71208401462959e-12 -1.34035709948127 -2.16263876278513;-2.9e-05 6.71455324269682e-12 -1.33954170864732 -2.16314391181559;-2.8e-05 6.71702151647629e-12 -1.33872612743462 -2.16364875341507;-2.7e-05 6.7194888356172e-12 -1.33791035595908 -2.1641532875118;-2.6e-05 6.72195519976888e-12 -1.33709439433664 -2.16465751403409;-2.5e-05 6.72442060858083e-12 -1.33627824268327 -2.16516143291027;-2.4e-05 6.72688506170264e-12 -1.33546190111496 -2.16566504406872;-2.3e-05 6.72934855878406e-12 -1.33464536974773 -2.16616834743787;-2.2e-05 6.73181109947497e-12 -1.33382864869763 -2.16667134294619;-2.1e-05 6.7342726834254e-12 -1.33301173808072 -2.16717403052219;-2e-05 6.73673331028549e-12 -1.33219463801313 -2.16767641009443;-1.9e-05 6.73919297970554e-12 -1.33137734861096 -2.16817848159151;-1.8e-05 6.74165169133597e-12 -1.33055986999038 -2.16868024494208;-1.7e-05 6.74410944482735e-12 -1.32974220226757 -2.16918170007481;-1.6e-05 6.74656623983037e-12 -1.32892434555874 -2.16968284691845;-1.5e-05 6.74902207599586e-12 -1.32810629998012 -2.17018368540177;-1.4e-05 6.75147695297481e-12 -1.32728806564798 -2.17068421545359;-1.3e-05 6.75393087041831e-12 -1.3264696426786 -2.17118443700278;-1.2e-05 6.75638382797761e-12 -1.32565103118831 -2.17168434997823;-1.1e-05 6.75883582530408e-12 -1.32483223129343 -2.1721839543089;-1e-05 6.76128686204926e-12 -1.32401324311036 -2.17268324992379;-9e-06 6.76373693786478e-12 -1.32319406675547 -2.17318223675194;-8e-06 6.76618605240244e-12 -1.32237470234519 -2.17368091472243;-7e-06 6.76863420531417e-12 -1.32155514999598 -2.17417928376438;-6e-06 6.77108139625202e-12 -1.32073540982431 -2.17467734380696;-5e-06 6.7735276248682e-12 -1.31991548194668 -2.1751750947794;-4e-06 6.77597289081504e-12 -1.31909536647963 -2.17567253661094;-3e-06 6.77841719374502e-12 -1.31827506353971 -2.1761696692309;-2e-06 6.78086053331075e-12 -1.3174545732435 -2.17666649256862;-1e-06 6.78330290916497e-12 -1.31663389570761 -2.17716300655348]  x5=5.70973484498186e-05  V1=ones(3,3)  V2=ones(3,3)  I1=ones(3,3)  I2=ones(3,3)  nHarmo=1  Measurements=None
  2-MW Load : powerlib/Elements/Three-Phase Parallel RLC Load  LConnTagsString=A|B|C  Configuration=Y (grounded)  NominalVoltage=25e3  Vabc=[1e3 1e3 1e3]  Vabcp=[1e3 1e3 1e3]  NominalFrequency=60  UnbalancedPower=off  ActivePower=2e6  InductivePower=0  CapacitivePower=0  Pabc=[10e3 9e3 11e3]  QLabc=[100 90 110]  QCabc=[100 90 110]  Pabcp=[10e3 9e3 11e3]  QLabcp=[100 90 110]  QCabcp=[100 90 110]  Measurements=None  LoadType=constant Z
  "3.3ohms " : powerlib/Elements/Series RLC Branch  LConnTagsString=__new0  RConnTagsString=__new0  BranchType=R  Resistance=3.3  Inductance=[]  SetiL0=off  InitialCurrent=0  Capacitance=[]  Setx0=off  InitialVoltage=0  Measurements=None
  30-MW 2-Mvar Load : powerlib/Elements/Three-Phase Parallel RLC Load  LConnTagsString=A|B|C  Configuration=Y (grounded)  NominalVoltage=25e3  Vabc=[1e3 1e3 1e3]  Vabcp=[1e3 1e3 1e3]  NominalFrequency=60  UnbalancedPower=off  ActivePower=30e6  InductivePower=2e6  CapacitivePower=0  Pabc=[10e3 9e3 11e3]  QLabc=[100 90 110]  QCabc=[100 90 110]  Pabcp=[10e3 9e3 11e3]  QLabcp=[100 90 110]  QCabcp=[100 90 110]  Measurements=None  LoadType=constant Z
  5-km Feeder : powerlib/Elements/Distributed Parameters Line  Phases=3  Frequency=60  Resistance=[0.1153 0.413]  Inductance=[1.05e-3 3.32e-3]  Capacitance=[11.33e-009 5.01e-009]  Length=5  x1=[-2.1e-05 -2.99808223273781e-09 -3537.1777559361 -24101.4118064339;-2e-05 -2.99763493458348e-09 -3528.09148660273 -24102.7435783266;-1.9e-05 -2.99718721039837e-09 -3519.00471584888 -24104.0719246818;-1.8e-05 -2.99673906024611e-09 -3509.91744496598 -24105.3968453109;-1.7e-05 -2.9962904841904e-09 -3500.82967524553 -24106.7183400255;-1.6e-05 -2.99584148229499e-09 -3491.74140797911 -24108.0364086378;-1.5e-05 -2.99539205462369e-09 -3482.65264445836 -24109.3510509605;-1.4e-05 -2.99494220124038e-09 -3473.56338597501 -24110.6622668067;-1.3e-05 -2.99449192220899e-09 -3464.47363382083 -24111.9700559901;-1.2e-05 -2.99404121759351e-09 -3455.38338928768 -24113.2744183248;-1.1e-05 -2.99359008745801e-09 -3446.29265366749 -24114.5753536254;-1e-05 -2.99313853186659e-09 -3437.20142825226 -24115.8728617071;-9e-06 -2.99268655088344e-09 -3428.10971433405 -24117.1669423855;-8e-06 -2.99223414457278e-09 -3419.017513205 -24118.4575954765;-7e-06 -2.99178131299892e-09 -3409.92482615731 -24119.7448207969;-6e-06 -2.99132805622622e-09 -3400.83165448325 -24121.0286181636;-5e-06 -2.99087437431908e-09 -3391.73799947518 -24122.3089873942;-4e-06 -2.990420267342e-09 -3382.64386242549 -24123.5859283067;-3e-06 -2.9899657353595e-09 -3373.54924462667 -24124.8594407197;-2e-06 -2.9895107784362e-09 -3364.45414737126 -24126.1295244521;-1e-06 -2.98905539663674e-09 -3355.35857195189 -24127.3961793234]  x2=[-2.1e-05 -3.05634567134866e-09 -3536.54260454984 -24100.0862322393;-2e-05 -3.05589579989161e-09 -3527.45683499129 -24101.4177647797;-1.9e-05 -3.05544549412361e-09 -3518.37056410246 -24102.7458719712;-1.8e-05 -3.05499475410866e-09 -3509.2837931747 -24104.0705536249;-1.7e-05 -3.05454357991083e-09 -3500.19652349946 -24105.3918095526;-1.6e-05 -3.05409197159424e-09 -3491.10875636822 -24106.7096395666;-1.5e-05 -3.05363992922306e-09 -3482.02049307258 -24108.0240434795;-1.4e-05 -3.05318745286155e-09 -3472.93173490417 -24109.3350211046;-1.3e-05 -3.05273454257401e-09 -3463.8424831547 -24110.6425722555;-1.2e-05 -3.05228119842481e-09 -3454.75273911597 -24111.9466967463;-1.1e-05 -3.05182742047839e-09 -3445.66250407983 -24113.2473943918;-1e-05 -3.05137320879922e-09 -3436.5717793382 -24114.5446650071;-9e-06 -3.05091856345187e-09 -3427.48056618309 -24115.8385084078;-8e-06 -3.05046348450096e-09 -3418.38886590654 -24117.12892441;-7e-06 -3.05000797201115e-09 -3409.2966798007 -24118.4159128303;-6e-06 -3.04955202604718e-09 -3400.20400915777 -24119.6994734858;-5e-06 -3.04909564667387e-09 -3391.11085527002 -24120.9796061942;-4e-06 -3.04863883395606e-09 -3382.01721942979 -24122.2563107734;-3e-06 -3.04818158795869e-09 -3372.92310292949 -24123.529587042;-2e-06 -3.04772390874673e-09 -3363.82850706159 -24124.7994348191;-1e-06 -3.04726579638523e-09 -3354.73343311865 -24126.0658539241]  x3=[-2.1e-05 -7.1577847997236e-12 -11.1569797667156 -79.1361781565402;-2e-05 -7.16027970415055e-12 -11.1271453382829 -79.1403786152132;-1.9e-05 -7.16277359094207e-12 -11.0973093284347 -79.1445678262735;-1.8e-05 -7.16526645974372e-12 -11.0674717414113 -79.1487457891256;-1.7e-05 -7.16775831020121e-12 -11.0376325814533 -79.1529125031759;-1.6e-05 -7.17024914196039e-12 -11.0077918528017 -79.1570679678319;-1.5e-05 -7.17273895466726e-12 -10.9779495596973 -79.1612121825033;-1.4e-05 -7.17522774796796e-12 -10.9481057063814 -79.1653451466011;-1.3e-05 -7.17771552150877e-12 -10.9182602970956 -79.1694668595377;-1.2e-05 -7.18020227493614e-12 -10.8884133360815 -79.1735773207275;-1.1e-05 -7.18268800789663e-12 -10.858564827581 -79.1776765295863;-1e-05 -7.18517272003697e-12 -10.8287147758363 -79.1817644855314;-9e-06 -7.18765641100402e-12 -10.7988631850897 -79.1858411879819;-8e-06 -7.19013908044481e-12 -10.7690100595838 -79.1899066363584;-7e-06 -7.19262072800647e-12 -10.7391554035614 -79.1939608300831;-6e-06 -7.19510135333632e-12 -10.7092992212656 -79.1980037685798;-5e-06 -7.19758095608181e-12 -10.6794415169395 -79.2020354512739;-4e-06 -7.20005953589052e-12 -10.6495822948265 -79.2060558775924;-3e-06 -7.20253709241021e-12 -10.6197215591705 -79.210065046964;-2e-06 -7.20501362528874e-12 -10.5898593142151 -79.2140629588188;-1e-06 -7.20748913417415e-12 -10.5599955642046 -79.2180496125887]  x4=[-2.1e-05 -9.43697225203683e-13 -12.5606320770324 -78.900076087335;-2e-05 -9.39649462396684e-13 -12.5308865572356 -78.9048057272276;-1.9e-05 -9.3560156604454e-13 -12.5011392565203 -78.9095241529875;-1.8e-05 -9.31553536722548e-13 -12.4713901791143 -78.9142313639442;-1.7e-05 -9.27505375006024e-13 -12.4416393292456 -78.9189273594288;-1.6e-05 -9.234570814703e-13 -12.4118867111426 -78.9236121387737;-1.5e-05 -9.19408656690731e-13 -12.3821323290336 -78.9282857013133;-1.4e-05 -9.15360101242687e-13 -12.3523761871475 -78.9329480463832;-1.3e-05 -9.11311415701559e-13 -12.3226182897132 -78.9375991733208;-1.2e-05 -9.07262600642755e-13 -12.2928586409601 -78.9422390814652;-1.1e-05 -9.03213656641702e-13 -12.2630972451176 -78.9468677701568;-1e-05 -8.99164584273845e-13 -12.2333341064155 -78.9514852387379;-9e-06 -8.95115384114647e-13 -12.2035692290838 -78.9560914865522;-8e-06 -8.91066056739591e-13 -12.1738026173527 -78.960686512945;-7e-06 -8.87016602724176e-13 -12.1440342754528 -78.9652703172633;-6e-06 -8.8296702264392e-13 -12.1142642076148 -78.9698428988557;-5e-06 -8.78917317074358e-13 -12.0844924180697 -78.9744042570722;-4e-06 -8.74867486591044e-13 -12.0547189110487 -78.9789543912645;-3e-06 -8.7081753176955e-13 -12.0249436907833 -78.9834933007862;-2e-06 -8.66767453185463e-13 -11.9951667615053 -78.9880209849919;-1e-06 -8.62717251414391e-13 -11.9653881274465 -78.9925374432383]  x5=2.03919101606495e-05  V1=ones(3,3)  V2=ones(3,3)  I1=ones(3,3)  I2=ones(3,3)  nHarmo=1  Measurements=None
  Ground3 : powerlib/Elements/Ground  LConnTagsString=a
  "Grounding Transformer " : powerlib/Elements/Grounding Transformer   UNITS=pu  NominalPower="[100e6   60]"  NominalVoltage=25e3  ZeroSequenceImpedance_pu=[0.025 0.75]  MagnetizationBranch_pu=[500 500]  ZeroSequenceImpedance_SI=[0.052083 589.05]  MagnetizationBranch_SI=[1041.7 3.927e+005]  Measurements=None
  A : PMIOPort  Port=1  Side=Left
  B : PMIOPort  Port=2  Side=Left
  C : PMIOPort  Port=3  Side=Left
  connections:
  "3.3ohms "/RConn1 -- Ground3/LConn1
  120 kV / 25 kV 47 MVA/LConn1 -- 120kV 2500MVA/RConn1
  120 kV / 25 kV 47 MVA/LConn2 -- 120kV 2500MVA/RConn2
  120 kV / 25 kV 47 MVA/LConn3 -- 120kV 2500MVA/RConn3
  120 kV / 25 kV 47 MVA/RConn1 -- "Grounding Transformer "/LConn1 -- 14-km Feeder/RConn1 -- 30-MW 2-Mvar Load/LConn1
  120 kV / 25 kV 47 MVA/RConn2 -- "Grounding Transformer "/LConn2 -- 14-km Feeder/RConn2 -- 30-MW 2-Mvar Load/LConn2
  120 kV / 25 kV 47 MVA/RConn3 -- "Grounding Transformer "/LConn3 -- 14-km Feeder/RConn3 -- 30-MW 2-Mvar Load/LConn3
  5-km Feeder/RConn1 -- 14-km Feeder/LConn1 -- 2-MW Load/LConn1
  5-km Feeder/RConn2 -- 14-km Feeder/LConn2 -- 2-MW Load/LConn2
  5-km Feeder/RConn3 -- 14-km Feeder/LConn3 -- 2-MW Load/LConn3
  A/RConn1 -- 5-km Feeder/LConn1
  B/RConn1 -- 5-km Feeder/LConn2
  C/RConn1 -- 5-km Feeder/LConn3
  "Grounding Transformer "/RConn1 -- "3.3ohms "/LConn1

== system power_PVarray_grid_det_LVRT/Irradiance Temp ==
  Demux : Demux  Tag=STV Demux  Outputs=2
  FromWs : FromWorkspace  Tag=STV FromWs  VariableName=tuvar  SampleTime=0  SigBuilderData=DataTag0  VnvData=DataTag1
      SigBuilderData=|
      | common.afterFinalStr = 'Extrapolate'
      | common.sampleTime = '0'
      | dataSet(1).timeRange = [0 2]
      | dataSet(1).name = 'Constant Irradiance'
      | dataSet(2).timeRange = [0 2]
      | dataSet(2).name = 'Step Irradiance'
      | dataSet(3).timeRange = [0 5]
      | dataSet(3).name = 'Ramp-up/down Irradiance'
      | sbobj.Groups(1).Name = 'Constant Irradiance'
      | sbobj.Groups(1).Signals(1).Name = 'Ir'
      | sbobj.Groups(1).Signals(1).XData = [0 2]
      | sbobj.Groups(1).Signals(1).YData = [1000 1000]
      | sbobj.Groups(1).Signals(2).Name = 'Temp'
      | sbobj.Groups(1).Signals(2).XData = [0 1 1 2]
      | sbobj.Groups(1).Signals(2).YData = [0 0 1 1]
      | sbobj.Groups(1).TimeRange = [0 2]
      | sbobj.Groups(2).Name = 'Step Irradiance'
      | sbobj.Groups(2).Signals(1).Name = 'Ir'
      | sbobj.Groups(2).Signals(1).XData = [0 0.252 0.252 2]
      | sbobj.Groups(2).Signals(1).YData = [600 600 1000 1000]
      | sbobj.Groups(2).Signals(2).Name = 'Temp'
      | sbobj.Groups(2).Signals(2).XData = [0 1 1 2]
      | sbobj.Groups(2).Signals(2).YData = [0 0 1 1]
      | sbobj.Groups(2).TimeRange = [0 2]
      | sbobj.Groups(3).Name = 'Ramp-up/down Irradiance'
      | sbobj.Groups(3).Signals(1).Name = 'Ir'
      | sbobj.Groups(3).Signals(1).XData = [0 0.6 1.1 1.2 1.7 5]
      | sbobj.Groups(3).Signals(1).YData = [1000 1000 1000 1000 1000 1000]
      | sbobj.Groups(3).Signals(2).Name = 'Temp'
      | sbobj.Groups(3).Signals(2).XData = [0 2 2.1 3 5]
      | sbobj.Groups(3).Signals(2).YData = [25 25 25 25 25]
      | sbobj.Groups(3).TimeRange = [0 5]
  Ir : Outport  Tag=STV Outport
  Temp : Outport  Tag=STV Outport  Port=2
  wires:
  Demux/1 -> Ir/1
  FromWs/1 -> Demux/1
  Demux/2 -> Temp/1

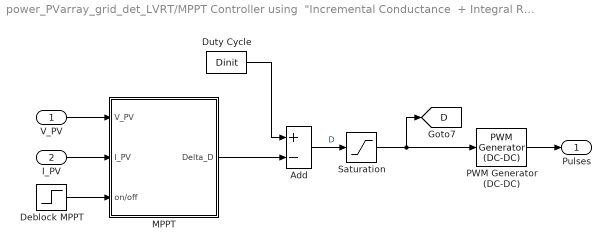
== system power_PVarray_grid_det_LVRT/MPPT Controller using  "Incremental Conductance  + Integral Regulator "  technique  ==
  V_PV : Inport
  I_PV : Inport  Port=2
  Add : Sum  Inputs=+-
  Deblock MPPT : Step  Time=0.4  SampleTime=0
  Duty Cycle : Constant  Value=Dinit
  MPPT : Subsystem
  PWM Generator (DC-DC) : powerlib_meascontrol/Pulse & Signal Generators/PWM Generator (DC-DC)  Fsw=fc  Ts=Ts_Power
  Saturation : Saturate  UpperLimit=1  LowerLimit=0
  Pulses : Outport
  tag scope: D=global
  wires:
  V_PV/1 -> MPPT/1(V_PV)
  I_PV/1 -> MPPT/2(I_PV)
  PWM Generator (DC-DC)/1 -> Pulses/1
  Deblock MPPT/1 -> MPPT/3(on/off)
  Saturation/1 -> PWM Generator (DC-DC)/1, [D]
  Add/1 -> Saturation/1  "D"
  MPPT/1(Delta_D) -> Add/2
  Duty Cycle/1 -> Add/1

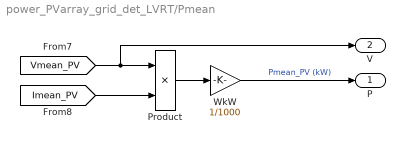
== system power_PVarray_grid_det_LVRT/Pmean ==
  Product : Product  RndMeth=Zero
  WkW : Gain  Gain=1/1000
  P : Outport
  V : Outport  Port=2
  wires:
  [Vmean_PV] -> Product/1, V/1
  Product/1 -> WkW/1
  [Imean_PV] -> Product/2
  WkW/1 -> P/1  "Pmean_PV (kW)"

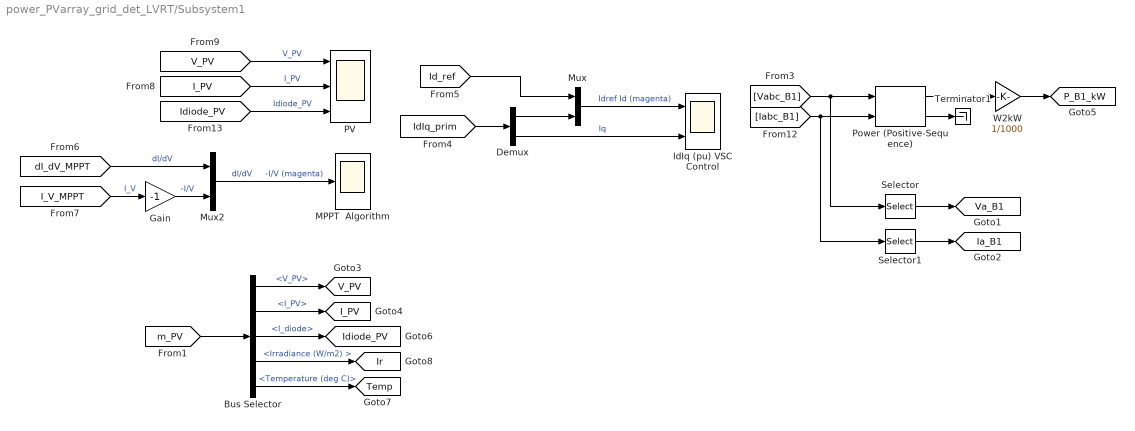
== system power_PVarray_grid_det_LVRT/Subsystem1 ==
  Bus Selector : BusSelector  OutputSignals=V_PV,I_PV,I_diode,Irradiance (W/m2) ,Temperature (deg C)
  Demux : Demux  Outputs=2
  Gain : Gain  Gain=-1
  IdIq (pu) VSC Control : Scope  NumInputPorts=2
  MPPT  Algorithm : Scope
  Mux : Mux  Inputs=2
  Mux2 : Mux  Inputs=2
  PV : Scope  NumInputPorts=3
  Power (Positive-Sequence) : powerlib_meascontrol/Measurements/Power (Positive-Sequence)  Freq=60  Vinit=[0, 0]  Iinit=[0, 0]  Ts=Ts_Control
  Selector : Selector  InputPortWidth=3  IndexOptions=Index vector (dialog)  Indices=[1]  OutputSizes=1
  Selector1 : Selector  InputPortWidth=3  IndexOptions=Index vector (dialog)  Indices=[1]  OutputSizes=1
  Terminator1 : Terminator
  W2kW : Gain  Gain=1/1000
  tag scope: I_PV=global, Ia_B1=global, Idiode_PV=global, Ir=global, P_B1_kW=global, Temp=global, V_PV=global, Va_B1=global
  wires:
  [Vabc_B1] -> Power (Positive-Sequence)/1, Selector/1
  [Iabc_B1] -> Power (Positive-Sequence)/2, Selector1/1
  Power (Positive-Sequence)/1 -> W2kW/1
  [I_V_MPPT] -> Gain/1  "I_V"
  [IdIq_prim] -> Demux/1
  [Id_ref] -> Mux/1
  Demux/1 -> Mux/2
  Mux/1 -> IdIq (pu) VSC Control/1  "Idref Id (magenta)"
  Demux/2 -> IdIq (pu) VSC Control/2  "Iq"
  Selector/1 -> [Va_B1]
  Selector1/1 -> [Ia_B1]
  [V_PV] -> PV/1  "V_PV"
  [I_PV] -> PV/2  "I_PV"
  [Idiode_PV] -> PV/3  "Idiode_PV"
  [dI_dV_MPPT] -> Mux2/1  "dI/dV"
  Gain/1 -> Mux2/2  "-I/V"
  Mux2/1 -> MPPT  Algorithm/1  "dI/dV     -I/V (magenta)"
  W2kW/1 -> [P_B1_kW]
  [m_PV] -> Bus Selector/1
  Bus Selector/1 -> [V_PV]  "<V_PV>"
  Bus Selector/2 -> [I_PV]  "<I_PV>"
  Bus Selector/4 -> [Ir]  "<Irradiance (W/m2) >"
  Bus Selector/3 -> [Idiode_PV]  "<I_diode>"
  Bus Selector/5 -> [Temp]  "<Temperature (deg C)>"
  Power (Positive-Sequence)/2 -> Terminator1/1

== system power_PVarray_grid_det_LVRT/Subsystem2 ==
  Mean : powerlib_meascontrol/Measurements/Mean  Freq=60  Vinit=0  Ts=Ts_Control
  Mux1 : Mux  Inputs=2
  Vm : Outport
  VrVm : Outport  Port=2
  wires:
  [Vdc_ref] -> Mux1/1  "Vdc ref"
  [Vdc] -> Mean/1  "Vdc"
  Mux1/1 -> VrVm/1
  Mean/1 -> Mux1/2, Vm/1

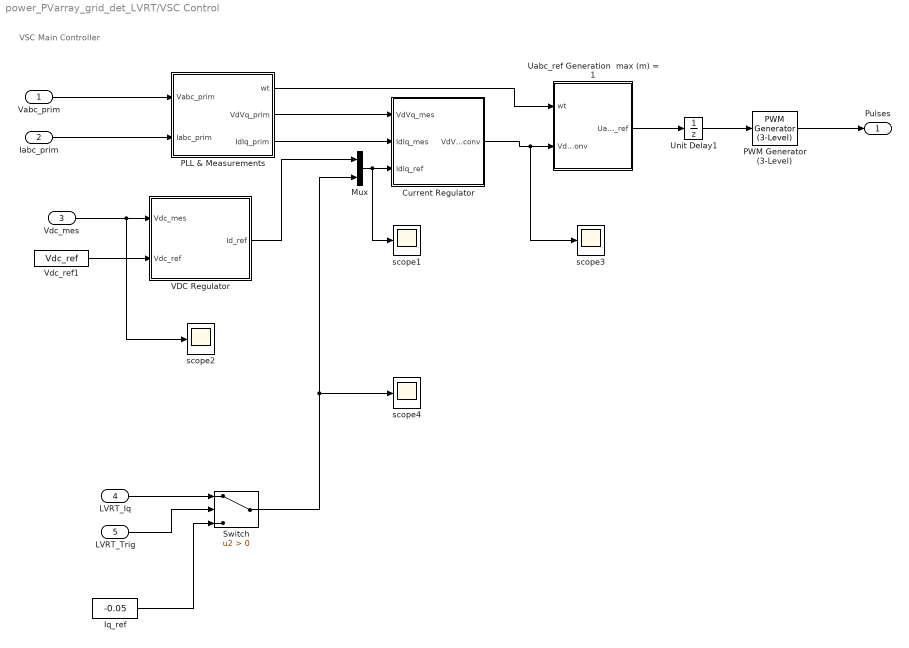
== system power_PVarray_grid_det_LVRT/VSC Control ==
  note: VSC Main Controller
  Vabc_prim : Inport  PortDimensions=3
  Iabc_prim : Inport  Port=2  PortDimensions=3
  Vdc_mes : Inport  Port=3  PortDimensions=1
  LVRT_Iq : Inport  Port=4
  LVRT_Trig : Inport  Port=5
  Current Regulator : Subsystem
  Iq_ref : Constant  Value=-0.05
  Mux : Mux  Inputs=2
  PLL & Measurements : Subsystem
  PWM Generator (3-Level) : powerlib_meascontrol/Pulse & Signal Generators/PWM Generator (3-Level)  ModulatorType=Three-phase bridge (12 pulses)  ModulatorMode=Unsynchronized  nF=27  Fc=33*60  ModulatingSignals=off  m=0.8  Freq=60  Phase=0  Ts=Ts_Power
  Switch : Switch  Criteria=u2 > Threshold
  Uabc_ref Generation  max (m) = 1 : Subsystem
  Unit Delay1 : UnitDelay  SampleTime=Ts_Control
  VDC Regulator : Subsystem
  Vdc_ref1 : Constant  Value=Vdc_ref
  scope{1..4} (4 alike) : Scope
  Pulses : Outport
  wires:
  VDC Regulator/1(Id_ref) -> Mux/1
  PLL & Measurements/1(wt) -> Uabc_ref Generation  max (m) = 1/1(wt)
  Current Regulator/1(VdVq_conv) -> scope3/1, Uabc_ref Generation  max (m) = 1/2(VdVq_conv)
  Mux/1 -> scope1/1, Current Regulator/3(IdIq_ref)
  PLL & Measurements/3(IdIq_prim) -> Current Regulator/2(IdIq_mes)
  PLL & Measurements/2(VdVq_prim) -> Current Regulator/1(VdVq_mes)
  Vdc_mes/1 -> scope2/1, VDC Regulator/1(Vdc_mes)
  Vabc_prim/1 -> PLL & Measurements/1(Vabc_prim)
  Iabc_prim/1 -> PLL & Measurements/2(Iabc_prim)
  Uabc_ref Generation  max (m) = 1/1(Uabc_ref) -> Unit Delay1/1
  PWM Generator (3-Level)/1 -> Pulses/1
  Vdc_ref1/1 -> VDC Regulator/2(Vdc_ref)
  Unit Delay1/1 -> PWM Generator (3-Level)/1
  LVRT_Iq/1 -> Switch/1
  LVRT_Trig/1 -> Switch/2
  Iq_ref/1 -> Switch/3
  Switch/1 -> scope4/1, Mux/2

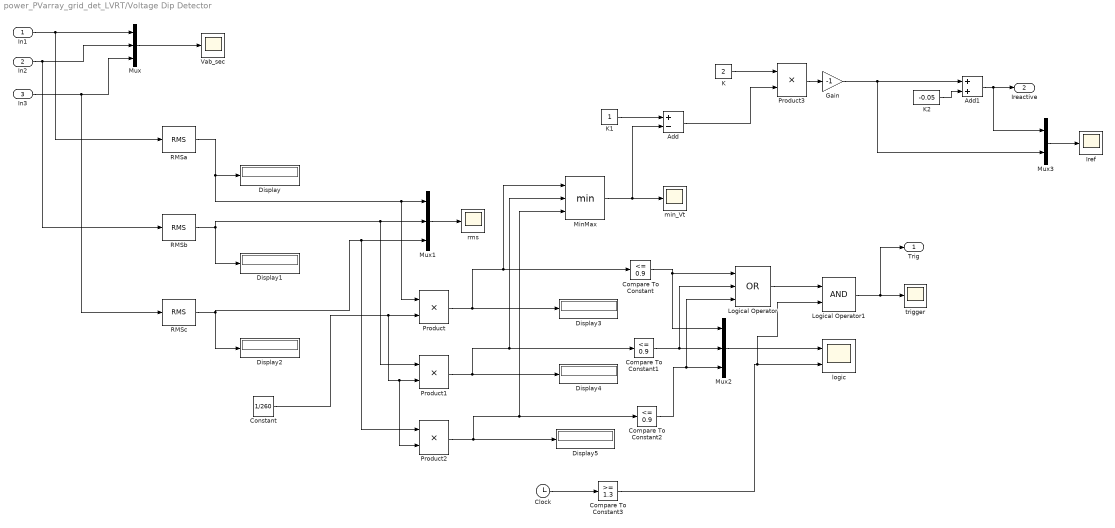
== system power_PVarray_grid_det_LVRT/Voltage Dip Detector ==
  In1 : Inport
  In2 : Inport  Port=2
  In3 : Inport  Port=3
  Add : Sum  Inputs=+-
  Add1 : Sum
  Clock : Clock
  Compare To Constant : simulink/Logic and Bit Operations/Compare To Constant  relop=<=  const=0.9  OutDataTypeStr=boolean
  Compare To Constant1 : simulink/Logic and Bit Operations/Compare To Constant  relop=<=  const=0.9  OutDataTypeStr=boolean
  Compare To Constant2 : simulink/Logic and Bit Operations/Compare To Constant  relop=<=  const=0.9  OutDataTypeStr=boolean
  Compare To Constant3 : simulink/Logic and Bit Operations/Compare To Constant  relop=>=  const=1.3  OutDataTypeStr=boolean
  Constant : Constant  Value=1/260
  Display{,1..5} (6 alike) : Display
  Gain : Gain  Gain=-1
  Iref : Scope
  K : Constant  Value=2
  K1 : Constant
  K2 : Constant  Value=-0.05
  Logical Operator : Logic  Operator=OR  Inputs=3  AllPortsSameDT=off  OutDataTypeStr=boolean
  Logical Operator1 : Logic  AllPortsSameDT=off  OutDataTypeStr=boolean
  MinMax : MinMax  Inputs=3
  Mux : Mux  Inputs=3
  Mux1 : Mux  Inputs=3
  Mux2 : Mux  Inputs=3
  Mux3 : Mux  Inputs=2
  Product{,1..3} (4 alike) : Product
  RMSa : powerlib_meascontrol/Measurements/RMS  TrueRMS=on  Freq=60  RMSInit=120  Ts=Ts_Power
  RMSb : powerlib_meascontrol/Measurements/RMS  TrueRMS=on  Freq=60  RMSInit=120  Ts=Ts_Power
  RMSc : powerlib_meascontrol/Measurements/RMS  TrueRMS=on  Freq=60  RMSInit=120  Ts=Ts_Power
  Vab_sec : Scope
  logic : Scope  NumInputPorts=2
  min_Vt : Scope
  rms : Scope
  trigger : Scope
  Trig : Outport
  Ireactive : Outport  Port=2
  wires:
  Mux/1 -> Vab_sec/1
  In1/1 -> RMSa/1, Mux/1
  In2/1 -> RMSb/1, Mux/2
  In3/1 -> RMSc/1, Mux/3
  RMSa/1 -> Product/1, Mux1/1, Display/1
  RMSb/1 -> Product1/1, Mux1/2, Display1/1
  RMSc/1 -> Product2/1, Mux1/3, Display2/1
  Mux1/1 -> rms/1
  Constant/1 -> Product2/2, Product1/2, Product/2
  Product/1 -> MinMax/1, Compare To Constant/1, Display3/1
  Product1/1 -> MinMax/2, Compare To Constant1/1, Display4/1
  Product2/1 -> MinMax/3, Compare To Constant2/1, Display5/1
  Clock/1 -> Compare To Constant3/1
  Compare To Constant/1 -> Logical Operator/1, Mux2/1
  Compare To Constant1/1 -> Logical Operator/2, Mux2/2
  Compare To Constant2/1 -> Logical Operator/3, Mux2/3
  Mux2/1 -> logic/1
  Logical Operator/1 -> Logical Operator1/1
  Compare To Constant3/1 -> Logical Operator1/2, logic/2
  Logical Operator1/1 -> Trig/1, trigger/1
  MinMax/1 -> Add/2, min_Vt/1
  K/1 -> Product3/1
  Product3/1 -> Gain/1
  K1/1 -> Add/1
  Add/1 -> Product3/2
  Gain/1 -> Mux3/2, Add1/1
  Add1/1 -> Mux3/1, Ireactive/1
  K2/1 -> Add1/2
  Mux3/1 -> Iref/1

== system power_PVarray_grid_det_LVRT/info ==

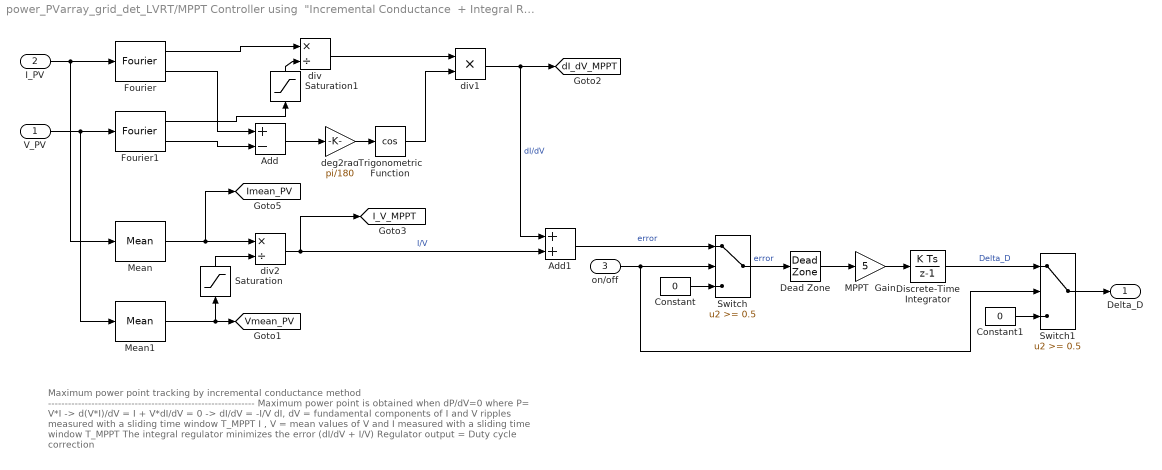
== system power_PVarray_grid_det_LVRT/MPPT Controller using  "Incremental Conductance  + Integral Regulator "  technique /MPPT ==
  note: Maximum power point tracking by incremental conductance method
      | --------------------------------------------------------------
      | Maximum power point is obtained when dP/dV=0  where P= V*I
      | -> d(V*I)/dV = I + V*dI/dV = 0
      | -> dI/dV = -I/V
      |
      | dI, dV  = fundamental components of I and V ripples measured with a sliding time window T_MPPT
      | I , V   = mean values of V and I measured with a sliding time window T_MPPT
      |
      | The integral regulator minimizes the error (dI/dV + I/V)
      | Regulator output = Duty cycle correction
  V_PV : Inport
  I_PV : Inport  Port=2
  on/off : Inport  Port=3
  Add : Sum  Inputs=+-
  Add1 : Sum
  Constant : Constant  Value=0
  Constant1 : Constant  Value=0
  Dead Zone : DeadZone  LowerValue=-0.05  UpperValue=0.05  SaturateOnIntegerOverflow=on
  Discrete-Time Integrator : DiscreteIntegrator  SampleTime=Ts_Control  LimitOutput=on  UpperSaturationLimit=1  LowerSaturationLimit=-1  ICPrevOutput=DiscIntNeverNeededParam  ICPrevScaledInput=DiscIntNeverNeededParam
  Fourier : powerlib_meascontrol/Measurements/Fourier  Freq=1/T_MPPT  n=1  InInit=[0, 0]  Ts=Ts_Control
  Fourier1 : powerlib_meascontrol/Measurements/Fourier  Freq=1/T_MPPT  n=1  InInit=[0, 0]  Ts=Ts_Control
  MPPT  Gain : Gain  Gain=5
  Mean : powerlib_meascontrol/Measurements/Mean  Freq=1/T_MPPT  Vinit=0  Ts=Ts_Control
  Mean1 : powerlib_meascontrol/Measurements/Mean  Freq=1/T_MPPT  Vinit=0  Ts=Ts_Control
  Saturation : Saturate  UpperLimit=inf  LowerLimit=eps
  Saturation1 : Saturate  UpperLimit=inf  LowerLimit=eps
  Switch : Switch  Threshold=0.5
  Switch1 : Switch  Threshold=0.5
  Trigonometric Function : Trigonometry  Operator=cos
  deg2rad : Gain  Gain=pi/180
  div : Product  Inputs=*/  RndMeth=Zero
  div1 : Product  Inputs=**  RndMeth=Zero
  div2 : Product  Inputs=*/  RndMeth=Zero
  Delta_D : Outport
  tag scope: I_V_MPPT=global, Imean_PV=global, Vmean_PV=global, dI_dV_MPPT=global
  wires:
  Dead Zone/1 -> MPPT  Gain/1
  Switch/1 -> Dead Zone/1  "error"
  Saturation1/1 -> div/2
  Saturation/1 -> div2/2
  Switch1/1 -> Delta_D/1
  on/off/1 -> Switch/2, Switch1/2
  Constant1/1 -> Switch1/3
  Discrete-Time Integrator/1 -> Switch1/1  "Delta_D"
  Constant/1 -> Switch/3
  MPPT  Gain/1 -> Discrete-Time Integrator/1
  Add1/1 -> Switch/1  "error"
  div2/1 -> Add1/2, [I_V_MPPT]  "I/V"
  Mean1/1 -> Saturation/1, [Vmean_PV]
  Mean/1 -> div2/1, [Imean_PV]
  div1/1 -> Add1/1, [dI_dV_MPPT]  "dI/dV"
  Trigonometric Function/1 -> div1/2
  div/1 -> div1/1
  deg2rad/1 -> Trigonometric Function/1
  Add/1 -> deg2rad/1
  Fourier1/1 -> Saturation1/1
  Fourier1/2 -> Add/2
  Fourier/2 -> Add/1
  V_PV/1 -> Mean1/1, Fourier1/1
  I_PV/1 -> Mean/1, Fourier/1
  Fourier/1 -> div/1
